simulink model "Simulation_articulatedVehicle"  (R2022a)
settings: Solver=ode15s  StartTime=0.0  StopTime=20  FixedStep=0.05  RelTol=1e-3
values from neighbouring files (symbols this model uses):
  alpha = deg2rad(20)    [main_articulatedVehicle.m]
  beta = deg2rad(15)    [main_articulatedVehicle.m]
  K = [lambda_1   lambda_2    0           0 ... (first row only)    [main_articulatedVehicle.m]
  l1 = 2    [main_articulatedVehicle.m]
  l2 = 3    [main_articulatedVehicle.m]
  max_dgamma = deg2rad(60)    [main_articulatedVehicle.m]
  max_gamma = deg2rad(45)    [main_articulatedVehicle.m]
  max_v = 15    [main_articulatedVehicle.m]
  min_dgamma = deg2rad(-60)    [main_articulatedVehicle.m]
  min_gamma = deg2rad(-45)    [main_articulatedVehicle.m]
  min_v = 0    [main_articulatedVehicle.m]
  q_hat0 = [xa_0 ya_0 thetaa_0 gamma_0 va_0]    [main_articulatedVehicle.m]
  timeStep = 0.005    [main_articulatedVehicle.m]
settings Model: Creator=Matteo Pettinari  LastModifiedBy=v
settings SolverCC: AlgebraicLoopSolver=TrustRegion
settings DebuggingCC: UnconnectedInputMsg=warning  UnconnectedOutputMsg=warning  UnconnectedLineMsg=warning  SFMachineParentedDataDiag=warning  ArithmeticOperatorsInVariantConditions=warning
settings SFSimCC: CustomCodeUndefinedFunction=UseInterfaceOnly
settings RTWCC: DLArmComputeVersion=19.05

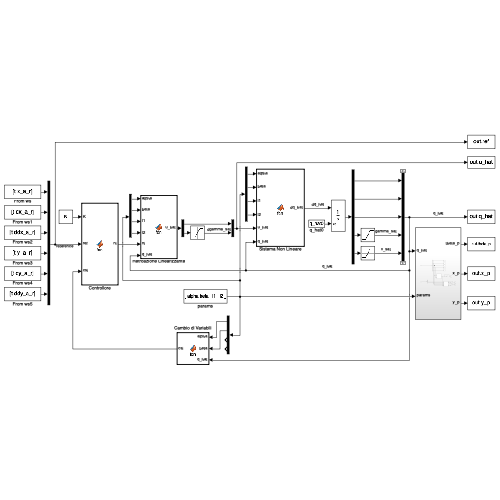
[thumbnail: Simulink's stored preview of the top-level diagram]
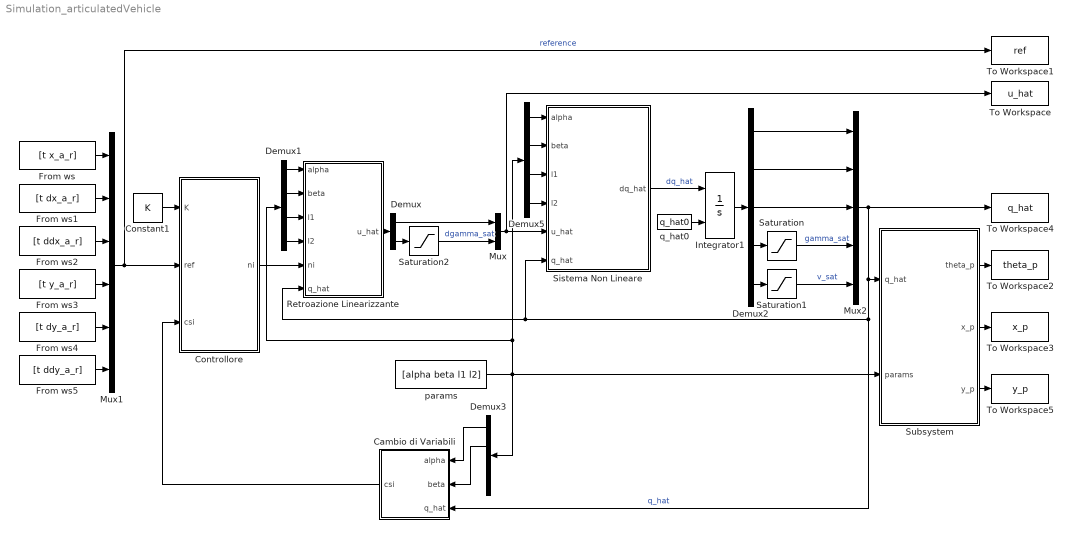
== system Simulation_articulatedVehicle ==
  Cambio di Variabili : MATLAB Function  TreatAsAtomicUnit=on
  Constant1 : Constant  Value=K
  Controllore : MATLAB Function  TreatAsAtomicUnit=on
  Demux : Demux  Outputs=2
  Demux1 : Demux
  Demux2 : Demux  Outputs=5
  Demux3 : Demux
  Demux5 : Demux
  From ws : FromWorkspace  VariableName=[t x_a_r]  SampleTime=timeStep
  From ws1 : FromWorkspace  VariableName=[t dx_a_r]  SampleTime=timeStep
  From ws2 : FromWorkspace  VariableName=[t ddx_a_r]  SampleTime=timeStep
  From ws3 : FromWorkspace  VariableName=[t y_a_r]  SampleTime=timeStep
  From ws4 : FromWorkspace  VariableName=[t dy_a_r]  SampleTime=timeStep
  From ws5 : FromWorkspace  VariableName=[t ddy_a_r]  SampleTime=timeStep
  Integrator1 : Integrator  InitialConditionSource=external
  Mux : Mux  Inputs=2
  Mux1 : Mux  Inputs=6
  Mux2 : Mux  Inputs=5
  Retroazione Linearizzante : MATLAB Function  TreatAsAtomicUnit=on
  Saturation : Saturate  UpperLimit=max_gamma  LowerLimit=min_gamma
  Saturation1 : Saturate  UpperLimit=max_v  LowerLimit=min_v
  Saturation2 : Saturate  UpperLimit=max_dgamma  LowerLimit=min_dgamma
  Sistema Non Lineare : MATLAB Function  TreatAsAtomicUnit=on
  Subsystem : Subsystem
  To Workspace : ToWorkspace  VariableName=u_hat  SaveFormat=Structure With Time  SampleTime=-1
  To Workspace1 : ToWorkspace  VariableName=ref  SaveFormat=Structure With Time
  To Workspace2 : ToWorkspace  VariableName=theta_p  SaveFormat=Structure With Time  SampleTime=-1
  To Workspace3 : ToWorkspace  VariableName=x_p  SaveFormat=Structure With Time  SampleTime=-1
  To Workspace4 : ToWorkspace  VariableName=q_hat  SaveFormat=Structure With Time  SampleTime=-1
  To Workspace5 : ToWorkspace  VariableName=y_p  SaveFormat=Structure With Time  SampleTime=-1
  params : Constant  Value=[alpha beta l1 l2]
  q_hat0 : Constant  Value=q_hat0
  wires:
  params/1 -> Demux5/1, Demux1/1, Subsystem/2(params), Demux3/1
  Constant1/1 -> Controllore/1(K)
  Cambio di Variabili/1(csi) -> Controllore/3(csi)
  Mux/1 -> Sistema Non Lineare/5(u_hat), To Workspace/1
  Demux1/2 -> Retroazione Linearizzante/2(beta)
  Demux3/2 -> Cambio di Variabili/2(beta)
  Demux1/1 -> Retroazione Linearizzante/1(alpha)
  Demux5/2 -> Sistema Non Lineare/2(beta)
  Demux1/3 -> Retroazione Linearizzante/3(l1)
  Demux1/4 -> Retroazione Linearizzante/4(l2)
  Demux5/3 -> Sistema Non Lineare/3(l1)
  Demux5/4 -> Sistema Non Lineare/4(l2)
  Demux5/1 -> Sistema Non Lineare/1(alpha)
  Demux3/1 -> Cambio di Variabili/1(alpha)
  Subsystem/2(x_p) -> To Workspace3/1
  Subsystem/3(y_p) -> To Workspace5/1
  Controllore/1(ni) -> Retroazione Linearizzante/5(ni)
  From ws/1 -> Mux1/1
  From ws4/1 -> Mux1/5
  From ws3/1 -> Mux1/4
  From ws2/1 -> Mux1/3
  From ws1/1 -> Mux1/2
  From ws5/1 -> Mux1/6
  Mux1/1 -> To Workspace1/1, Controllore/2(ref)  "reference"
  Subsystem/1(theta_p) -> To Workspace2/1
  Demux2/4 -> Saturation/1
  Sistema Non Lineare/1(dq_hat) -> Integrator1/1  "dq_hat"
  q_hat0/1 -> Integrator1/2
  Integrator1/1 -> Demux2/1
  Demux2/2 -> Mux2/2
  Demux2/1 -> Mux2/1
  Saturation/1 -> Mux2/4  "gamma_sat"
  Saturation1/1 -> Mux2/5  "v_sat"
  Demux2/5 -> Saturation1/1
  Mux2/1 -> Cambio di Variabili/3(q_hat), Retroazione Linearizzante/6(q_hat), Sistema Non Lineare/6(q_hat), Subsystem/1(q_hat), To Workspace4/1  "q_hat"
  Demux2/3 -> Mux2/3
  Demux/2 -> Saturation2/1
  Saturation2/1 -> Mux/2  "dgamma_sat"
  Demux/1 -> Mux/1
  Retroazione Linearizzante/1(u_hat) -> Demux/1

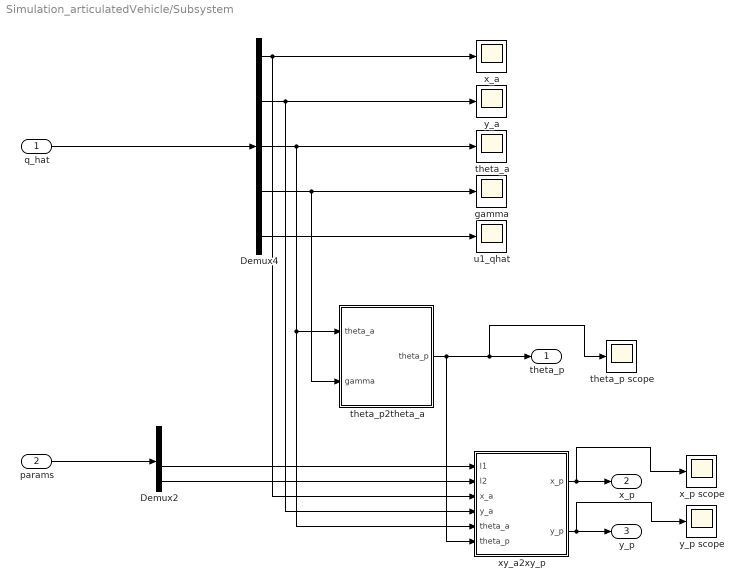
== system Simulation_articulatedVehicle/Subsystem ==
  q_hat : Inport
  params : Inport  Port=2
  Demux2 : Demux
  Demux4 : Demux  Outputs=5
  gamma : Scope
  theta_a : Scope
  theta_p scope : Scope
  theta_p2theta_a : MATLAB Function  TreatAsAtomicUnit=on
  u1_qhat : Scope
  x_a : Scope
  x_p scope : Scope
  xy_a2xy_p : MATLAB Function  TreatAsAtomicUnit=on
  y_a : Scope
  y_p scope : Scope
  theta_p : Outport
  x_p : Outport  Port=2
  y_p : Outport  Port=3
  wires:
  Demux2/4 -> xy_a2xy_p/2(l2)
  Demux4/1 -> x_a/1, xy_a2xy_p/3(x_a)
  params/1 -> Demux2/1
  theta_p2theta_a/1(theta_p) -> theta_p/1, theta_p scope/1, xy_a2xy_p/6(theta_p)
  q_hat/1 -> Demux4/1
  Demux4/4 -> gamma/1, theta_p2theta_a/2(gamma)
  xy_a2xy_p/1(x_p) -> x_p scope/1, x_p/1
  Demux4/2 -> y_a/1, xy_a2xy_p/4(y_a)
  xy_a2xy_p/2(y_p) -> y_p scope/1, y_p/1
  Demux2/3 -> xy_a2xy_p/1(l1)
  Demux4/3 -> theta_a/1, theta_p2theta_a/1(theta_a), xy_a2xy_p/5(theta_a)
  Demux4/5 -> u1_qhat/1

== matlab function Simulation_articulatedVehicle/Cambio di Variabili ==
  data: alpha input; beta input; csi output; q_hat input
function csi = fcn(alpha, beta, q_hat)

% Spacchetto lo stato
x1 = q_hat(1);
x2 = q_hat(2);
x3 = q_hat(3);
x4 = q_hat(4);
u1 = q_hat(5);


% Cambio coordinate
csi = [x1; ...
       u1 * cos(x3 + beta); ...
       x2; ...
       u1 * sin(x3 + beta)];

end

== matlab function Simulation_articulatedVehicle/Controllore ==
  data: K input; ni output; ref input; csi input
function ni = fcn(K, ref, csi)

ni = zeros(2, 1);

% Spacchetto il riferimento
xr      = ref(1);
dxr     = ref(2);
ddxr    = ref(3);
yr      = ref(4);
dyr     = ref(5);
ddyr    = ref(6);


y_ref   = [ddxr;
           ddyr];
err     = [csi(1) - xr;
           csi(2) - dxr;
           csi(3) - yr;
           csi(4) - dyr];

% Legge di controllo
ni = y_ref - K * err;
            
end

== matlab function Simulation_articulatedVehicle/Retroazione Linearizzante ==
  data: alpha input; beta input; l1 input; l2 input; ni input; q_hat input; u_hat output
function u_hat = fcn(alpha, beta, l1, l2, ni, q_hat)

u_hat = zeros(2, 1);

% Spacchetto lo stato
x1 = q_hat(1);
x2 = q_hat(2);
x3 = q_hat(3);
x4 = q_hat(4);
u1 = q_hat(5);


E = [cos(beta + x3), -(l2*u1*sin(beta + x3)*cos(alpha))/(l2*cos(alpha) + l1*cos(alpha - x4));
     sin(beta + x3),  (l2*u1*cos(beta + x3)*cos(alpha))/(l2*cos(alpha) + l1*cos(alpha - x4))];

Gamma = [(u1^2*(cos(2*beta - alpha + x3 + x4) - cos(alpha + x3 - x4)))/(2*l2*cos(alpha) + 2*l1*cos(alpha - x4));
         (u1^2*(sin(2*beta - alpha + x3 + x4) - sin(alpha + x3 - x4)))/(2*l2*cos(alpha) + 2*l1*cos(alpha - x4))];

% Ingresso fisico
u_hat = -E \ (Gamma - ni);


end

== matlab function Simulation_articulatedVehicle/Sistema Non Lineare ==
  data: alpha input; beta input; l1 input; l2 input; u_hat input; q_hat input; dq_hat output
function dq_hat = fcn(alpha, beta, l1, l2, u_hat, q_hat)

dq_hat = zeros(5, 1);

% Spacchetto lo stato
x1 = q_hat(1);
x2 = q_hat(2);
x3 = q_hat(3);
x4 = q_hat(4);
x5 = q_hat(5);


% Forma affine di controllo
f = [x5 * cos(x3 + beta);
     x5 * sin(x3 + beta);
     x5 * sin(x4 + beta - alpha)/(l1 * cos(x4 - alpha) + l2 * cos(alpha));
     0;
     0];

g_1 = [0;
       0;
       0;
       0;
       1];
 
g_2 = [0;
       0;
       l2 * cos(alpha)/(l1 * cos(x4 - alpha) + l2 * cos(alpha));
       1;
       0];

g = [g_1    g_2];


% Dinamica
dq_hat = f + g * u_hat;

end

== matlab function Simulation_articulatedVehicle/Subsystem/theta_p2theta_a ==
  data: theta_a input; gamma input; theta_p output
function theta_p = fcn(theta_a, gamma)

theta_p = theta_a - gamma;

end

== matlab function Simulation_articulatedVehicle/Subsystem/xy_a2xy_p ==
  data: l1 input; l2 input; x_a input; y_a input; x_p output; theta_a input; theta_p input; y_p output
function [x_p, y_p] = fcn(l1, l2, x_a, y_a, theta_a, theta_p)

x_p = x_a - l1 * cos(theta_a) - l2 * cos(theta_p);
y_p = y_a - l1 * sin(theta_a) - l2 * sin(theta_p);

end
